simulink model "pure_pursuit_2"  (R2015b)
settings: Solver=FixedStepDiscrete  StartTime=0.0  StopTime=10  FixedStep=0.01  RelTol=1e-3
settings Model: Creator=castiel_liu  LastModifiedBy=castiel_liu

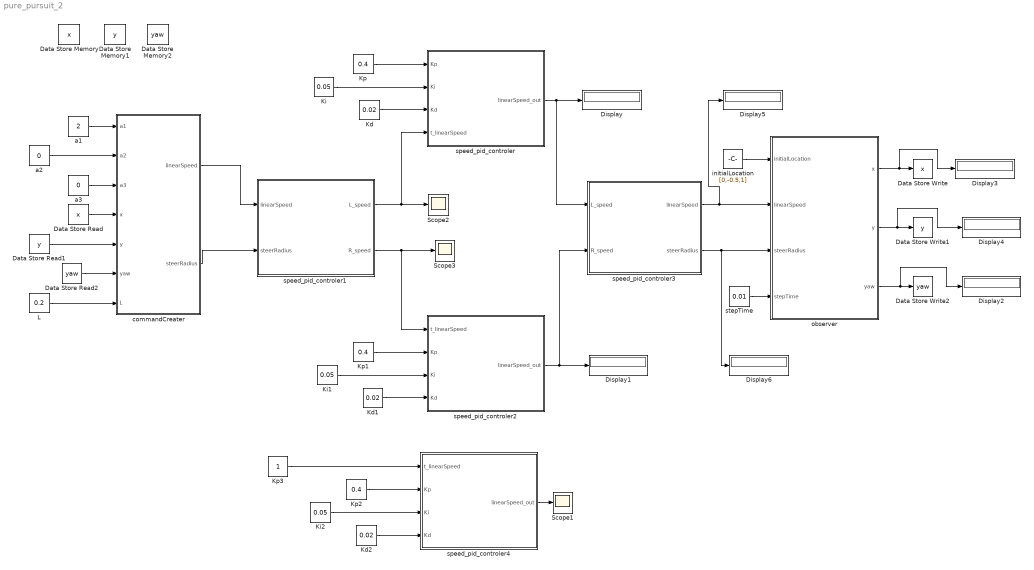
== system pure_pursuit_2 ==
  Data Store Memory : DataStoreMemory  DataStoreName=x  ReadBeforeWriteMsg=warning  WriteAfterWriteMsg=warning  WriteAfterReadMsg=warning
  Data Store Memory1 : DataStoreMemory  DataStoreName=y  ReadBeforeWriteMsg=warning  WriteAfterWriteMsg=warning  WriteAfterReadMsg=warning
  Data Store Memory2 : DataStoreMemory  DataStoreName=yaw  ReadBeforeWriteMsg=warning  WriteAfterWriteMsg=warning  WriteAfterReadMsg=warning
  Data Store Read : DataStoreRead  DataStoreName=x
  Data Store Read1 : DataStoreRead  DataStoreName=y
  Data Store Read2 : DataStoreRead  DataStoreName=yaw
  Data Store Write : DataStoreWrite  DataStoreName=x
  Data Store Write1 : DataStoreWrite  DataStoreName=y
  Data Store Write2 : DataStoreWrite  DataStoreName=yaw
  Display{,1..6} (7 alike) : Display
  Kd : Constant  Value=0.02
  Kd1 : Constant  Value=0.02
  Kd2 : Constant  Value=0.02
  Ki : Constant  Value=0.05
  Ki1 : Constant  Value=0.05
  Ki2 : Constant  Value=0.05
  Kp : Constant  Value=0.4
  Kp1 : Constant  Value=0.4
  Kp2 : Constant  Value=0.4
  Kp3 : Constant
  L : Constant  Value=0.2
  Scope1 : Scope
  Scope2 : Scope
  Scope3 : Scope
  a1 : Constant  Value=2
  a2 : Constant  Value=0
  a3 : Constant  Value=0
  commandCreater : MATLAB Function  TreatAsAtomicUnit=on
  initialLocation : Constant  Value=[0,-0.5,1]
  "observer " : MATLAB Function  TreatAsAtomicUnit=on
  speed_pid_controler : MATLAB Function  TreatAsAtomicUnit=on
  speed_pid_controler1 : MATLAB Function  TreatAsAtomicUnit=on
  speed_pid_controler2 : MATLAB Function  TreatAsAtomicUnit=on
  speed_pid_controler3 : MATLAB Function  TreatAsAtomicUnit=on
  speed_pid_controler4 : MATLAB Function  TreatAsAtomicUnit=on
  stepTime : Constant  Value=0.01
  wires:
  stepTime/1 -> "observer "/4(stepTime)
  commandCreater/2(steerRadius) -> speed_pid_controler1/2(steerRadius)
  L/1 -> commandCreater/7(L)
  "observer "/2(y) -> Display4/1, Data Store Write1/1
  "observer "/1(x) -> Display3/1, Data Store Write/1
  Data Store Read/1 -> commandCreater/4(x)
  Data Store Read1/1 -> commandCreater/5(y)
  Data Store Read2/1 -> commandCreater/6(yaw)
  "observer "/3(yaw) -> Display2/1, Data Store Write2/1
  a2/1 -> commandCreater/2(a2)
  a3/1 -> commandCreater/3(a3)
  a1/1 -> commandCreater/1(a1)
  initialLocation/1 -> "observer "/1(initialLocation)
  Kd/1 -> speed_pid_controler/3(Kd)
  Ki/1 -> speed_pid_controler/2(Ki)
  Kp/1 -> speed_pid_controler/1(Kp)
  speed_pid_controler/1(linearSpeed_out) -> Display/1, speed_pid_controler3/1(L_speed)
  speed_pid_controler1/1(L_speed) -> Scope2/1, speed_pid_controler/4(t_linearSpeed)
  commandCreater/1(linearSpeed) -> speed_pid_controler1/1(linearSpeed)
  Kd1/1 -> speed_pid_controler2/4(Kd)
  Ki1/1 -> speed_pid_controler2/3(Ki)
  Kp1/1 -> speed_pid_controler2/2(Kp)
  speed_pid_controler1/2(R_speed) -> Scope3/1, speed_pid_controler2/1(t_linearSpeed)
  speed_pid_controler2/1(linearSpeed_out) -> Display1/1, speed_pid_controler3/2(R_speed)
  speed_pid_controler3/1(linearSpeed) -> Display5/1, "observer "/2(linearSpeed)
  speed_pid_controler3/2(steerRadius) -> Display6/1, "observer "/3(steerRadius)
  Kd2/1 -> speed_pid_controler4/4(Kd)
  Ki2/1 -> speed_pid_controler4/3(Ki)
  Kp2/1 -> speed_pid_controler4/2(Kp)
  Kp3/1 -> speed_pid_controler4/1(t_linearSpeed)
  speed_pid_controler4/1(linearSpeed_out) -> Scope1/1

== matlab function pure_pursuit_2/observer  ==
  data: initialLocation input; linearSpeed input; x output; steerRadius input; y output; stepTime input; yaw output
function [x,y,yaw] = fcn(initialLocation,linearSpeed,steerRadius,stepTime)
%#左转时转弯半径为负数
persistent x0;
persistent y0;
persistent theta0;
persistent first_time_flag;

if(isempty(x0))
    x0 = 0;
    y0 = 0;
    theta0 = 0.0;
    first_time_flag = 1;
end

fp = fopen('record.txt','a');
if(first_time_flag == 1)
    x=initialLocation(1);
    y=initialLocation(2);
    yaw = initialLocation(3);
    first_time_flag = 0;
else
    angularSpeed = linearSpeed / (steerRadius);

    theta = angularSpeed * stepTime;
    alpha = theta/2;
    if(alpha ~=0)
        rho = 2*steerRadius*sin(alpha); 
    else
        rho = linearSpeed * stepTime;
    end
    %旋转坐标变换矩阵
    convertMatrix = [cos(theta0),sin(theta0);-sin(theta0),cos(theta0)];

    temp = convertMatrix * [rho*cos(alpha),rho*sin(alpha)]'+[x0;y0];
    x = temp(1);
    y = temp(2);
    yaw = -( theta0+theta);
end

x0 = x;
y0 = y;
theta0 =-yaw;
    

fprintf(fp,'%f\t%f\n',x,y); 
fprintf('%f\t%f\t%f\n',x,y,yaw);
fclose(fp);


end

== matlab function pure_pursuit_2/speed_pid_controler ==
  data: Kp input; Ki input; linearSpeed_out output; Kd input; t_linearSpeed input
function linearSpeed_out = fcn(Kp,Ki,Kd,t_linearSpeed)
persistent last_err
persistent last_last_err
persistent sigma_err
persistent last_val %上一次的值

if(isempty(last_err))
    last_err = 0;
    sigma_err = 0;
    last_val =0;
    last_last_err=0;
end 

err = t_linearSpeed - last_val;
sigma_err = sigma_err + err;
linearSpeed_out = Kp *err +Ki*sigma_err +Kd* (err-last_err);
%linearSpeed_out = Kp*(err-last_err) +Ki*err +Kd*(err-2*last_err+last_last_err);
last_last_err = last_err;
last_err = err;
last_val = linearSpeed_out;

%fprintf('%f\t%f\t%f\n',err,linearSpeed_out,sigma_err);
end

== matlab function pure_pursuit_2/commandCreater ==
  data: a1 input; a2 input; a3 input; linearSpeed output; steerRadius output; x input; y input; yaw input; L input
function [linearSpeed,steerRadius] = fcn(a1,a2,a3,x,y,yaw,L)
persistent target_x;
persistent target_y;
persistent last_linear_speed;
if(isempty(target_x))
    target_x = 0;
    last_linear_speed = 0;
end
% if(isempty(target_y))
%     target_y = 0;
% end
%左转时转弯半径为负数

target_y = a1*target_x + a2*target_x^2 + a3*target_x^3;
%target_y = sin(target_x);
dis = (target_y-y)^2+(target_x-x)^2;
t_yaw = atan2(target_y-y,target_x-x);
if(dis < L*L)
    target_x = target_x +0.01;
    linearSpeed = last_linear_speed;
    steerRadius = inf;
    %fprintf('linearSpeed= %f\tsteerRadius=%f\n',linearSpeed,steerRadius);
else
    linearSpeed = 1;
    steerRadius = -sqrt(dis)/(2*sin(t_yaw-yaw));
    if(steerRadius >10) 
        steerRadius=inf;
    end
end
%fprintf('dis=%f\n',dis);
last_linear_speed = linearSpeed;

%fprintf('%f\t%f\t%f\t%f\t%f\t%f\t%f\n',t_yaw*180/pi,yaw*180/pi,steerRadius,linearSpeed, sqrt(dis),target_x,target_y);
end

== matlab function pure_pursuit_2/speed_pid_controler1 ==
  data: linearSpeed input; steerRadius input; L_speed output; R_speed output
function [L_speed,R_speed] = fcn(linearSpeed,steerRadius)
    WHEEL_BASE = 0.5; %轮距0.5m
    angularSpeed = linearSpeed/steerRadius;
    L_speed = linearSpeed + (angularSpeed * WHEEL_BASE)/2;
    R_speed = linearSpeed - (angularSpeed * WHEEL_BASE)/2;

== matlab function pure_pursuit_2/speed_pid_controler2 ==
  data: t_linearSpeed input; Kp input; Ki input; linearSpeed_out output; Kd input
function linearSpeed_out = fcn(t_linearSpeed,Kp,Ki,Kd)
persistent last_err
persistent last_last_err
persistent sigma_err
persistent last_val %上一次的值

if(isempty(last_err))
    last_err = 0;
    sigma_err = 0;
    last_val =0;
    last_last_err=0;
end 

err = t_linearSpeed - last_val;
sigma_err = sigma_err + err;
linearSpeed_out = Kp *err +Ki*sigma_err +Kd* (err-last_err);
%linearSpeed_out = Kp*(err-last_err) +Ki*err +Kd*(err-2*last_err+last_last_err);
last_last_err = last_err;
last_err = err;
last_val = linearSpeed_out;

%fprintf('%f\t%f\t%f\n',err,linearSpeed_out,sigma_err);
end

== matlab function pure_pursuit_2/speed_pid_controler3 ==
  data: linearSpeed output; steerRadius output; L_speed input; R_speed input
function [linearSpeed,steerRadius] = fcn(L_speed,R_speed)
    WHEEL_BASE = 0.5; %轮距0.5m
    if(L_speed == R_speed)
        steerRadius = Inf;
    else
        steerRadius = WHEEL_BASE*(L_speed+R_speed)/(L_speed-R_speed)/2;
    end
    linearSpeed = (L_speed+R_speed)/2;

== matlab function pure_pursuit_2/speed_pid_controler4 ==
  data: t_linearSpeed input; Kp input; Ki input; linearSpeed_out output; Kd input
function linearSpeed_out = fcn(t_linearSpeed,Kp,Ki,Kd)
persistent last_err
persistent last_last_err
persistent sigma_err
persistent last_val %上一次的值

if(isempty(last_err))
    last_err = 0;
    sigma_err = 0;
    last_val =0;
    last_last_err=0;
end 

err = t_linearSpeed - last_val;
sigma_err = sigma_err + err;
linearSpeed_out = Kp *err +Ki*sigma_err +Kd* (err-last_err);
%linearSpeed_out = Kp*(err-last_err) +Ki*err +Kd*(err-2*last_err+last_last_err);
last_last_err = last_err;
last_err = err;
last_val = linearSpeed_out;

%fprintf('%f\t%f\t%f\n',err,linearSpeed_out,sigma_err);
end
